simulink subsystem "repetitive_control"  (R2022b)
settings: Solver=VariableStepAuto  StartTime=0.0  StopTime=10.0  RelTol=1e-3
model mask{Np=0, N1=0, N2=0, Fzpet_num=0, Fzpet_den=0, Q_coe=0, Qzpet_num=0, Qzpet_den=0}
  mask prompts: Np "Number of Samples in a Period"; N1 "Plant Relative Degree + ZPET Degree"; N2 "ZPLPF Degree"; Fzpet_num "Fzpet Numerator"; Fzpet_den "Fzpet Denominator"; Q_coe "Q Coefficients"; Qzpet_num "Q Num"; Qzpet_den "Q Den"
undefined symbols (not defined in the file or in its folder): Ts
settings Model: Creator=Alex Zhen  LastModifiedBy=Alex Zhen

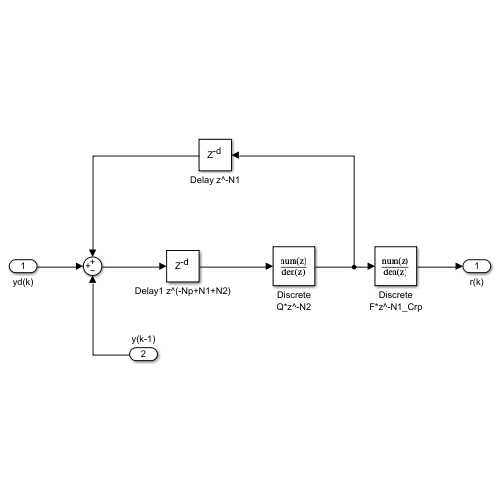
[thumbnail: Simulink's stored preview of the top-level diagram]
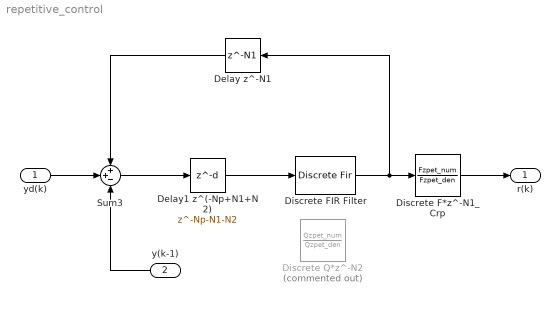
== system repetitive_control ==
  yd(k) : Inport
  y(k-1) : Inport  Port=2
  Delay z^-N1 : Delay  DelayLength=N1
  Delay1 z^(-Np+N1+N2) : Delay  DelayLength=Np-N1-N2
  Discrete F*z^-N1_Crp : DiscreteTransferFcn  Numerator=Fzpet_num  Denominator=Fzpet_den  SampleTime=Ts
  Discrete Q*z^-N2 : DiscreteTransferFcn  Commented=on  Numerator=Qzpet_num  Denominator=Qzpet_den  SampleTime=Ts
  Discrete FIR Filter : DiscreteFir  Coefficients=Q_coe
  Sum3 : Sum  Inputs=++-
  r(k) : Outport
  wires:
  Delay z^-N1/1 -> Sum3/1
  y(k-1)/1 -> Sum3/3
  Sum3/1 -> Delay1 z^(-Np+N1+N2)/1
  yd(k)/1 -> Sum3/2
  Discrete F*z^-N1_Crp/1 -> r(k)/1
  Delay1 z^(-Np+N1+N2)/1 -> Discrete FIR Filter/1
  Discrete FIR Filter/1 -> Discrete F*z^-N1_Crp/1, Delay z^-N1/1
